simulink model "reference_angle"  (R2013b)
settings: Solver=ode45  StartTime=0.0  StopTime=10.0  MaxStep=0.001  RelTol=1e-3
settings Model: Creator=aberger  LastModifiedBy=aberger
settings DataIOCC: MaxDataPoints=10000

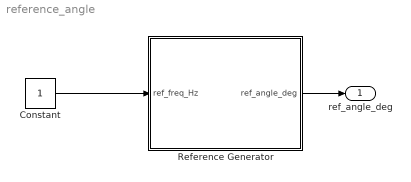
== system reference_angle ==
  Constant : Constant
  Reference Generator : Subsystem
  ref_angle_deg : Outport
  wires:
  Reference Generator/1(ref_angle_deg) -> ref_angle_deg/1
  Constant/1 -> Reference Generator/1(ref_freq_Hz)

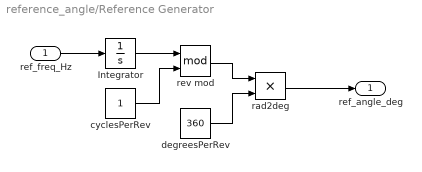
== system reference_angle/Reference Generator ==
  ref_freq_Hz : Inport
  Integrator : Integrator
  cyclesPerRev : Constant
  degreesPerRev : Constant  Value=360
  rad2deg : Product
  rev mod : Math  Operator=mod  SaturateOnIntegerOverflow=on
  ref_angle_deg : Outport
  wires:
  ref_freq_Hz/1 -> Integrator/1
  rad2deg/1 -> ref_angle_deg/1
  rev mod/1 -> rad2deg/1
  Integrator/1 -> rev mod/1
  degreesPerRev/1 -> rad2deg/2
  cyclesPerRev/1 -> rev mod/2
